simulink library "tire"  (R2020b)
settings: Solver=VariableStepAuto  StartTime=0.0  StopTime=10.0  RelTol=1e-3
undefined symbols (not defined in the file): Brakes_caliperD, Brakes_effectiveR, Brakes_kineticMu, Brakes_pads_front, Brakes_staticMu, Rim_mass, Tire_Cg, Tire_Cx, Tire_Cy, Tire_Lx, Tire_Ly, Tire_mass, Tire_muMax, Tire_muMin, Tire_prs_front, Tire_radius, Tire_VerticalK, Wheel_inertia, Wheel_width, X, Y, Z
libraries: nesl_utility x26, sm_lib x22, vehdynlibtire x2
(part 1 of 3)
settings Model: Creator=Adri  LastModifiedBy=Adri

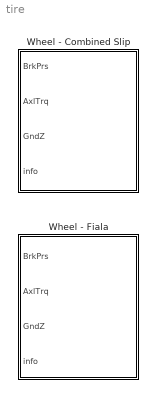
== system tire ==
  Wheel - Combined Slip : Subsystem  mask{side=Left, sideSign=1, Brake_staticMu=Brakes_staticMu, Brake_kineticMu=Brakes_kineticMu, Brake_actuatorD=Brakes_caliperD, Brake_effectiveR=Brakes_effectiveR, Brake_pads=Brakes_pads_front, Tire_radius=Tire_radius, Wheel_width=Wheel_width, Wheel_mass=Tire_mass + Rim_mass, Wheel_inertia=Wheel_inertia, Tire_prs=Tire_prs_front, Tire_verticalStiffness=Tire_VerticalK}
      mask prompts: Brake_staticMu "Static friction coefficient"; Brake_kineticMu "Kinetic friction coefficient"; Brake_actuatorD "Caliper actuator diameter"; Brake_effectiveR "Brake effective radius"; Brake_pads "Number of brake pads"; Tire_radius "Unloaded tire radius"; Wheel_width "Wheel width"; Wheel_mass "Wheel mass"; Wheel_inertia "Wheel inertia"; Tire_prs "Inflation pressure"; Tire_verticalStiffness "Vertical tire stiffness"
      settings: PortSchema="{\"entries\":[{\"content\":{\"sides\":[{\"content\":{\"connectorIds\":[\"LConn1\"]},\"type\":\"ConnectorPlacement.EquallySpacedRectSide\",\"uuid\":\"3662be25-634c-4dcf-b299-b3e3ad14fab2\"},{\"content\":{\"connectorIds\":[\"In1\",\"In2\",\"In3\",\"Out1\"],\"side\":\"RIGHT\"},\"type\":\"ConnectorPlacement.EquallySpacedRectSide\",\"uuid\":\"5eeeefc2-deff-4d04-aaf6-b6ca9cb4dfd2\"},{\"content\":{\"connectorIds\":[],\"side\":\"TOP\"},\"type\":\"ConnectorPlacement.EquallySpacedRectSide\",\"uuid\":\"9d9babff-f6dc-4e3d-b7b9-f7737e3c7694\"},{\"content\":{\"connectorIds\":[\"RConn1\"],\"side\":\"BOTTOM\"},\"type\":\"ConnectorPlacement.EquallySpacedRectSide\",\"uuid\":\"502eca10-01c6-46bc-9936-4bbe633b06d6\"}]},\"type\":\"ConnectorPlacement.EquallySpacedConnector\",\"uuid\":\"66182f26-71c7-4d18-82ec-2eaaaae22dab\"}],\"packageUris\":[\"http://schema.mathworks.com/mf0/Connector/19700101\"],\"version\":\"1.0\"}"
      mask TypeOptions side: Left | Right
      mask Callback side:
      | switch get_param(gcb,'side')
      |     case 'Left'
      |         set_param(gcb,'sideSign','1');
      |     case 'Right'
      |         set_param(gcb,'sideSign','-1');
      | end
      mask DialogControl DescGroupVar Prompt: Wheel
      mask DialogControl Container5 Prompt: Brakes
      mask DialogControl Brake_actuatorD Tooltip: (mm)
      mask DialogControl Brake_effectiveR Tooltip: (mm)
      mask DialogControl Container6 Prompt: Tires
      mask DialogControl Tire_radius Tooltip: (mm)
      mask DialogControl Wheel_width Tooltip: (mm)
      mask DialogControl Wheel_mass Tooltip: (kg)
      mask DialogControl Wheel_inertia Tooltip: (kg*m^2)
      mask DialogControl Tire_prs Tooltip: (Pa)
      mask DialogControl Tire_verticalStiffness Tooltip: (N/m)
      mask Display: image('$imagefile'); % Use "Edit Image" on toolstrip to change.
  Wheel - Fiala : Subsystem  mask{side=Left, sideSign=1, Brake_staticMu=Brakes_staticMu, Brake_kineticMu=Brakes_kineticMu, Brake_actuatorD=Brakes_caliperD, Brake_effectiveR=Brakes_effectiveR, Brake_pads=Brakes_pads_front, Tire_Cx=Tire_Cx, Tire_Cy=Tire_Cy, Tire_Cg=Tire_Cg, Tire_muKinetic=Tire_muMin, Tire_muStatic=Tire_muMax, Tire_Lx=Tire_Lx, Tire_Ly=Tire_Ly, Tire_radius=Tire_radius, Wheel_inertia=Wheel_inertia, Tire_Rdamp=0, Wheel_width=Wheel_width, Wheel_mass=Tire_mass + Rim_mass, Tire_prs=Tire_prs_front, Tire_Kz=Tire_VerticalK}
      mask prompts: Brake_staticMu "Static friction coefficient"; Brake_kineticMu "Kinetic friction coefficient"; Brake_actuatorD "Caliper actuator diameter"; Brake_effectiveR "Brake effective radius"; Brake_pads "Number of brake pads"; Tire_Cx "Longitudinal stiffness"; Tire_Cy "Lateral stiffness"; Tire_Cg "Camber stiffness"; Tire_muKinetic "Kinematic friction"; Tire_muStatic "Static friction"; Tire_Lx "Longitudinal relaxation length"; Tire_Ly "Lateral relaxation length"; Tire_radius "Unloaded tire radius"; Wheel_inertia "Wheel rotational inertia"; Tire_Rdamp "Rotational damping"; Wheel_width "Wheel width"; Wheel_mass "Wheel mass"; Tire_prs "Inflation pressure"; Tire_Kz "Vertical tire stiffness"
      settings: PortSchema="{\"entries\":[{\"content\":{\"sides\":[{\"content\":{\"connectorIds\":[\"LConn1\"]},\"type\":\"ConnectorPlacement.EquallySpacedRectSide\",\"uuid\":\"3662be25-634c-4dcf-b299-b3e3ad14fab2\"},{\"content\":{\"connectorIds\":[\"In1\",\"In2\",\"In3\",\"Out1\"],\"side\":\"RIGHT\"},\"type\":\"ConnectorPlacement.EquallySpacedRectSide\",\"uuid\":\"5eeeefc2-deff-4d04-aaf6-b6ca9cb4dfd2\"},{\"content\":{\"connectorIds\":[],\"side\":\"TOP\"},\"type\":\"ConnectorPlacement.EquallySpacedRectSide\",\"uuid\":\"9d9babff-f6dc-4e3d-b7b9-f7737e3c7694\"},{\"content\":{\"connectorIds\":[\"RConn1\"],\"side\":\"BOTTOM\"},\"type\":\"ConnectorPlacement.EquallySpacedRectSide\",\"uuid\":\"502eca10-01c6-46bc-9936-4bbe633b06d6\"}]},\"type\":\"ConnectorPlacement.EquallySpacedConnector\",\"uuid\":\"66182f26-71c7-4d18-82ec-2eaaaae22dab\"}],\"packageUris\":[\"http://schema.mathworks.com/mf0/Connector/19700101\"],\"version\":\"1.0\"}"
      mask TypeOptions side: Left | Right
      mask Callback side:
      | switch get_param(gcb,'side')
      |     case 'Left'
      |         set_param(gcb,'sideSign','1');
      |     case 'Right'
      |         set_param(gcb,'sideSign','-1');
      | end
      mask DialogControl DescGroupVar Prompt: Wheel
      mask DialogControl Container5 Prompt: Brakes
      mask DialogControl Brake_actuatorD Tooltip: (mm)
      mask DialogControl Brake_effectiveR Tooltip: (mm)
      mask DialogControl Container6 Prompt: Tires
      mask DialogControl Container7 Prompt: Longitudinal and lateral
      mask DialogControl Tire_Cx Tooltip: (N)
      mask DialogControl Tire_Cy Tooltip: (N/rad)
      mask DialogControl Tire_Cg Tooltip: (N/rad)
      mask DialogControl Tire_Lx Tooltip: (m)
      mask DialogControl Tire_Ly Tooltip: (m)
      mask DialogControl Container8 Prompt: Rolling
      mask DialogControl Tire_radius Tooltip: (mm)
      mask DialogControl Wheel_inertia Tooltip: (kg*m^2)
      mask DialogControl Tire_Rdamp Tooltip: (N*m)/(rad/s)
      mask DialogControl Container12 Prompt: Aligning
      mask DialogControl Wheel_width Tooltip: (mm)
      mask DialogControl Container11 Prompt: Vertical
      mask DialogControl Wheel_mass Tooltip: (kg)
      mask DialogControl Tire_prs Tooltip: (Pa)
      mask DialogControl Tire_Kz Tooltip: (N/m)
      mask Display: image('$imagefile'); % Use "Edit Image" on toolstrip to change.

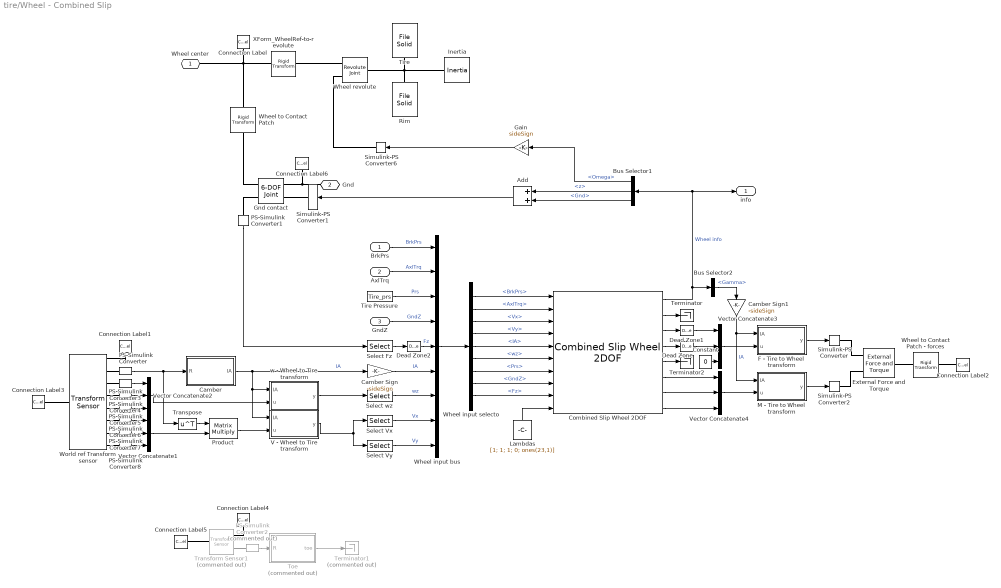
== system tire/Wheel - Combined Slip ==
  BrkPrs : Inport
  AxlTrq : Inport  Port=2
  GndZ : Inport  Port=3
  Add : Sum
  Bus Selector1 : BusSelector  OutputSignals=Omega,z,Gnd
  Bus Selector2 : BusSelector  OutputSignals=Gamma
  Camber : MATLAB Function  TreatAsAtomicUnit=on
  Camber Sign : Gain  Gain=-sideSign
  Camber Sign1 : Gain  Gain=-sideSign
  Combined Slip Wheel 2DOF : vehdynlibtire/Combined Slip Wheel 2DOF  BrakeType=Disc  mu_static=Brake_staticMu  mu_kinetic=Brake_kineticMu  disk_abore=Brake_actuatorD*1e-3  Rm=Brake_effectiveR*1e-3  num_pads=Brake_pads  drum_abore=0.0508  drum_a=0.123  drum_c=0.212  drum_r=0.15  drum_theta1=0  drum_theta2=126  brake_p_bpt=[1 11.4736842105263 21.9473684210526 32.4210526315789 42.8947368421053 53.3684210526316 63.8421052631579 74.3157894736842 84.7894736842105 95.2631578947368 105.736842105263 116.210526315789 126.684210526316 137.157894736842 147.631578947368 158.105263157895 168.578947368421 179.052631578947 189.526315789474 200]  brake_n_bpt=[0 52.6315789473684 105.263157894737 157.894736842105 210.526315789474 263.157894736842 315.789473684211 368.421052631579 421.052631578947 473.684210526316 526.315789473684 578.947368421053 631.578947368421 684.210526315789 736.842105263158 789.473684210526 842.105263157895 894.736842105263 947.368421052632 1000]  f_brake_t=[43.4900602404453 42.5056030554862 41.5350898940194 40.5780454442085 39.6340111501808 38.7025443887544 37.7832176914519 36.8756180088306 35.9793460143796 35.0940154454303 34.2192524787115 33.3546951383474 32.4999927342521 31.6548053290159 30.8188032315107 29.991666515561 29.1730845621415 28.362755623661 27.5603864089927 26.765691687993;498.991217495636 487.695866636631 476.560505099801 465.579679307235 454.748127933653 444.060772460445 433.51270824929 423.099196101319 412.81565427025 402.657650900201 392.620896861006 382.701238955775 372.894653477208 363.197240090814 353.605216024701 344.114910546964 334.722759712992 325.425301366216 316.219170376863 307.10109410434;954.492374750826 932.886130217776 911.585920305583 890.581313170261 869.862244717126 849.419000532136 829.242198807128 809.322774193808 789.651962526121 770.221286354971 751.0225412433 732.047782773203 713.289314220164 694.739674852612 676.391628817892 658.238154578366 640.272434863842 622.48784710877 604.877954344734 587.436496520688;1409.99353200602 1378.07639379892 1346.61133551136 1315.58294703329 1284.9763615006 1254.77722860383 1224.97168936497 1195.5463522863 1166.48827078199 1137.78492180974 1109.42418562559 1081.39432659063 1053.68397496312 1026.28210961441 999.178041611083 972.361398609768 945.822110014692 919.550392851325 893.536738312604 867.771898937035;1865.49468926121 1823.26665738007 1781.63675071715 1740.58458089631 1700.09047828407 1660.13545667552 1620.7011799228 1581.76993037878 1543.32457903786 1505.34855726451 1467.82583000789 1430.74087040806 1394.07863570608 1357.82454437621 1321.96445440427 1286.48464264117 1251.37178516554 1216.61293859388 1182.19552228048 1148.10730135338;2320.9958465164 2268.45692096121 2216.66216592293 2165.58621475934 2115.20459506754 2065.49368474721 2016.43067048064 1967.99350847127 1920.16088729373 1872.91219271928 1826.22747439018 1780.08741422549 1734.47329644903 1689.36697913801 1644.75086719747 1600.60788667257 1556.92146031639 1513.67548433643 1470.85430624835 1428.44270376973;2776.49700377159 2713.64718454235 2651.68758112871 2590.58784862237 2530.31871185102 2470.8519128189 2412.16016103848 2354.21708656376 2296.9971955496 2240.47582817405 2184.62911877248 2129.43395804292 2074.86795719199 2020.9094138998 1967.53727999066 1914.73113070398 1862.47113546724 1810.73803007899 1759.51309021622 1708.77810618608;3231.99816102678 3158.8374481235 3086.71299633449 3015.58948248539 2945.43282863449 2876.21014089059 2807.88965159632 2740.44066465625 2673.83350380547 2608.03946362882 2543.03076315477 2478.78050186034 2415.26261793494 2352.4518486616 2290.32369278385 2228.85437473538 2168.02081061809 2107.80057582154 2048.17187418409 1989.11350860242;3687.49931828197 3604.02771170464 3521.73841154027 3440.59111634842 3360.54694541796 3281.56836896228 3203.61914215416 3126.66424274874 3050.66981206134 2975.60309908359 2901.43240753707 2828.12704567777 2755.6572786779 2683.9942834234 2613.11010557704 2542.97761876678 2473.57048576894 2404.8631215641 2336.83065815196 2269.44891101877;4143.00047553716 4049.21797528579 3956.76382674606 3865.59275021144 3775.66106220143 3686.92659703397 3599.34863271199 3512.88782084123 3427.50612031721 3343.16673453836 3259.83405191936 3177.4735894952 3096.05193942085 3015.5367181852 2935.89651837023 2857.10086279818 2779.12016091979 2701.92566730665 2625.48944211983 2549.78431343512;4598.50163279235 4494.40823886693 4391.78924195184 4290.59438407447 4190.77517898491 4092.28482510566 3995.07812326983 3899.11139893372 3804.34242857308 3710.73036999313 3618.23569630166 3526.82013331263 3436.44660016381 3347.079152947 3258.68293116342 3171.22410682959 3084.66983607064 2998.98821304921 2914.1482260877 2830.11971585147;5054.00279004754 4939.59850244808 4826.81465715762 4715.59601793749 4605.88929576838 4497.64305317735 4390.80761382767 4285.3349770262 4181.17873682896 4078.2940054479 3976.63734068395 3876.16667713006 3776.84126090677 3678.62158770879 3581.46934395661 3485.34735086099 ...(+2764 chars)]  tireParamSet=vdynPassCar.mat  plySteer=off  turnslip=off  PRESMAX=1003118  PRESMIN=9982  FZMAX=3500  FZMIN=100  VXLOW=0.5  KPUMAX=2  KPUMIN=-2  ALPMAX=1.5708  ALPMIN=-1.5708  CAMMAX=0.173142086627737  CAMMIN=-0.173348165334087  LONGVL=16.7  omegao=0  br=1e-3  UNLOADED_RADIUS=Tire_radius*1e-3  NOMPRES=1e5  FNOMIN=750  WIDTH=Wheel_width*1e-3  RIM_RADIUS=.19  MASS=Wheel_mass  IYY=Wheel_inertia(3)  GRAVITY=-9.80665  zo=0  zdoto=0  BREFF=8.25094594147963  DREFF=0.260468730454265  FREFF=0.0735298544471851  Q_RE0=1.00866439868088  Q_V1=0.000760413786224011  Q_V2=0.0463384792019201  Q_FZ1=0  Q_FZ2=15.6870832810226  Q_FZ3=0  Q_FCX=0.138643970247602  Q_FCY=0.10843499565426  Q_FCY2=-0.465763352339538  PFZ1=0.69958166705601  VERTICAL_STIFFNESS=Tire_verticalStiffness  VERTICAL_DAMPING=494.649255786991  BOTTOM_OFFST=.01  BOTTOM_STIFF=2e6  LONGITUDINAL_STIFFNESS=388714.175879854  LATERAL_STIFFNESS=157087.404633332  PCFX1=0.18539229191199  PCFX2=0  PCFX3=0  PCFY1=0.163183345037677  PCFY2=0  PCFY3=0.249094918231954  Q_RA1=0.675942571700787  Q_RA2=0.73800463546164  Q_RB1=1.04487486456705  Q_RB2=-1.191763806629  PCX1=1.58523057950359  PDX1=1.0239116238178  PDX2=-0.0842405110022724  PDX3=0  PEX1=0.110312777158455  PEX2=0.313468516038146  PEX3=0  PEX4=0.0016060905760045  PKX1=21.3872544684023  PKX2=14.0006541873175  PKX3=-0.405326109653452  PHX1=0.000212599305364818  PHX2=0.00115950515263055  PVX1=1.59236164471432e-05  PVX2=0.000104321112127671  PPX1=-0.349461321276586  PPX2=0.387840040616429  PPX3=-0.0969947336569324  PPX4=0.0632271859795801  RBX1=12.7633329850276  RBX2=9.5787123658471  RBX3=0  RCX1=1.02796280922059  REX1=-0.45202516851367  REX2=-0.47304886171176  RHX1=0.000233272373115809  QSX1=-0.00788307788961443  QSX2=0.954629515459396  QSX3=0.0155855777667025  QSX4=0.125904607142414  QSX5=1.01110069703963  QSX6=20.1938577118433  QSX7=0.310818120717083  QSX8=-0.0430823751139655  QSX9=0.636494404888216  QSX10=0.142438060591663  QSX11=0.346766530036373  QSX12=0  QSX13=0  QSX14=0  PPMX1=0  PCY1=1.34299950037631  PDY1=0.878267729082195  PDY2=-0.0644597923147385  PDY3=0  PEY1=-0.809776534470972  PEY2=-0.600180598867198  PEY3=0.0991732552633487  PEY4=-6.5577974035573  PEY5=0  PKY1=-15.5714726518315  PKY2=1.73126522291751  PKY3=0.365349873517229  PKY4=1.98176755955416  PKY5=0  PKY6=-0.884005199550313  PKY7=-0.237259727611847  PHY1=-0.00183370557235628  PHY2=0.00346401302716671  PVY1=-0.00675427560163264  PVY2=0.036379218103843  PVY3=-0.163543984089166  PVY4=-0.491003349625726  PPY1=-0.62059646553185  PPY2=-0.0647824842338686  PPY3=-0.164648843290686  PPY4=0.283193909060098  PPY5=0  RBY1=10.7588809173639  RBY2=7.70420065295029  RBY3=3.40283755070691e-06  RBY4=0  RCY1=1.06691874059059  REY1=0.308244924574305  REY2=7.48775032604508e-06  RHY1=0.0118479204960415  RHY2=7.63650177161071e-06  RVY1=0.0560024425050078  RVY2=7.48487127056197e-06  RVY3=0  RVY4=98.4047026517149  RVY5=2.02759273900054  RVY6=15.7623064923347  QSY1=0.00699077564863536  QSY2=0  QSY3=0.00153535478298811  QSY4=8.55710322455322e-05  QSY5=0  QSY6=0  QSY7=0.89443879773793  QSY8=-0.403227641260894  QBZ1=11.666656027484  QBZ2=-1.30355438574485  QBZ3=0  QBZ4=0.177918305399071  QBZ5=-0.162481135068033  QBZ6=0  QBZ9=30.1445534682089  QBZ10=0  QCZ1=1.29026978207574  QDZ1=0.0886972644991399  QDZ2=-0.0058634820161856  QDZ3=0.3805597481383  QDZ4=0  QDZ6=0.00160914918118959  QDZ7=-0.00211036330862154  QDZ8=-0.13921904912557  QDZ9=0.00816585550028243  QDZ10=0  QDZ11=0  QEZ1=-2.19802254534746  QEZ2=1.01850535789165  QEZ3=0  QEZ4=0.278379679112054  QEZ5=-0.548414722765386  QHZ1=0.00148361198869669  QHZ2=0.00202017567585904  QHZ3=0.240316641332066  QHZ4=-0.210114035738085  PPZ1=-0.443927982388615  PPZ2=0  SSZ1=0.00914999585397887  SSZ2=0.0389830656052735  SSZ3=0  SSZ4=0  PDXP1=0.396718274678791  PDXP2=0  PDXP3=0  PKYP1=1.00587060633573  PDYP1=0.40483048923438  PDYP2=0  PDYP3=0  PDYP4=0  PHYP1=0.992731942067188  PHYP2=0.150352945499914  PHYP3=0  PHYP4=-3.98988682633674  PECP1=0.502379254513503  PECP2=0  QDTP1=10.0178654287947  QCRP1=0.200627747200702  QCRP2=0.0995735881599772  QBRP1=0.0997107127960717  QDRP1=1.01432910167423  QDRP2=0  aMode=2
      link override Magic Tire Const Input/Fx Relaxation/Integrator: AbsoluteTolerance=1e-2
      link override Magic Tire Const Input/Fy Relaxation/Integrator: AbsoluteTolerance=1e-2
      link override Magic Tire Const Input/My Relaxation/Integrator: AbsoluteTolerance=1e-2
      settings: SourceProductBaseCode=VE
  Connection Label{,1..2,4} (4 alike) : ConnectionLabel  Label=WheelRef
  Connection Label3 : ConnectionLabel  Label=GroundRef
  Connection Label5 : ConnectionLabel  Label=ChassisRef
  Connection Label6 : ConnectionLabel  Label=GroundRef
  Constant : Constant  Value=0
  Dead Zone : DeadZone  LowerValue=-10  UpperValue=10  ZeroCross=off  SaturateOnIntegerOverflow=on
  Dead Zone1 : DeadZone  LowerValue=-1  UpperValue=1  ZeroCross=off  SaturateOnIntegerOverflow=on
  Dead Zone2 : DeadZone  LowerValue=-inf  UpperValue=0  ZeroCross=off  SaturateOnIntegerOverflow=on
  External Force and Torque : sm_lib/Forces and Torques/External Force and Torque  ForceResolutionFrame=AttachedFrame  EnableForceX=off  EnableForceY=off  EnableForceZ=off  EnableForce=on  TorqueResolutionFrame=AttachedFrame  EnableTorqueX=off  EnableTorqueY=off  EnableTorqueZ=off  EnableTorque=on
  F - Tire to Wheel transform : MATLAB Function  TreatAsAtomicUnit=on
  Gain : Gain  Gain=sideSign
  Gnd contact : sm_lib/Joints/6-DOF Joint  JointMode=Normal  SenseConstraintForce=off  SenseConstraintForceX=off  SenseConstraintForceY=off  SenseConstraintForceZ=off  SenseConstraintTorque=off  SenseConstraintTorqueX=off  SenseConstraintTorqueY=off  SenseConstraintTorqueZ=off  SenseTotalForce=on  SenseTotalForceX=off  SenseTotalForceY=off  SenseTotalForceZ=off  SenseTotalTorque=off  SenseTotalTorqueX=off  SenseTotalTorqueY=off  SenseTotalTorqueZ=off  CompositeWrenchDir=BaseOnFollower  CompositeWrenchFrame=BaseFrame  PxEquilibriumPosition=0  PxEquilibriumPositionUnits=m  PxSpringStiffness=0  PxSpringStiffnessUnits=N/m  PxDampingCoefficient=0  PxDampingCoefficientUnits=N/(m/s)  PxTorqueActuationMode=NoTorque  PxMotionActuationMode=ComputedMotion  PxSensePosition=off  PxSenseVelocity=off  PxSenseAcceleration=off  PxSenseTorqueForce=off  PxSenseLowerLimitTorqueForce=off  PxSenseUpperLimitTorqueForce=off  PxLowerLimitSpecify=off  PxLowerLimitBound=-1  PxLowerLimitBoundUnits=m  PxLowerLimitStiffness=1e6  PxLowerLimitStiffnessUnits=N/m  PxLowerLimitDamping=1e3  PxLowerLimitDampingUnits=N/(m/s)  PxLowerLimitTransitionRegionWidth=1e-4  PxLowerLimitTransitionRegionWidthUnits=m  PxUpperLimitSpecify=off  PxUpperLimitBound=1  PxUpperLimitBoundUnits=m  PxUpperLimitStiffness=1e6  PxUpperLimitStiffnessUnits=N/m  PxUpperLimitDamping=1e3  PxUpperLimitDampingUnits=N/(m/s)  PxUpperLimitTransitionRegionWidth=1e-4  PxUpperLimitTransitionRegionWidthUnits=m  PxPositionTargetSpecify=off  PxPositionTargetPriority=Low  PxPositionTargetValue=-500  PxPositionTargetValueUnits=mm  PxVelocityTargetSpecify=off  PxVelocityTargetPriority=High  PxVelocityTargetValue=0  PxVelocityTargetValueUnits=m/s  PyEquilibriumPosition=0  PyEquilibriumPositionUnits=m  PySpringStiffness=0  PySpringStiffnessUnits=N/m  PyDampingCoefficient=0  PyDampingCoefficientUnits=N/(m/s)  PyTorqueActuationMode=NoTorque  PyMotionActuationMode=ComputedMotion  PySensePosition=off  PySenseVelocity=off  PySenseAcceleration=off  PySenseTorqueForce=off  PySenseLowerLimitTorqueForce=off  PySenseUpperLimitTorqueForce=off  PyLowerLimitSpecify=off  PyLowerLimitBound=-1  PyLowerLimitBoundUnits=m  PyLowerLimitStiffness=1e6  PyLowerLimitStiffnessUnits=N/m  PyLowerLimitDamping=1e3  PyLowerLimitDampingUnits=N/(m/s)  PyLowerLimitTransitionRegionWidth=1e-4  PyLowerLimitTransitionRegionWidthUnits=m  PyUpperLimitSpecify=off  PyUpperLimitBound=1  PyUpperLimitBoundUnits=m  PyUpperLimitStiffness=1e6  PyUpperLimitStiffnessUnits=N/m  PyUpperLimitDamping=1e3  PyUpperLimitDampingUnits=N/(m/s)  PyUpperLimitTransitionRegionWidth=1e-4  PyUpperLimitTransitionRegionWidthUnits=m  PyPositionTargetSpecify=off  PyPositionTargetPriority=Low  PyPositionTargetValue=600*sideSign  PyPositionTargetValueUnits=mm  PyVelocityTargetSpecify=off  PyVelocityTargetPriority=High  PyVelocityTargetValue=0  PyVelocityTargetValueUnits=m/s  PzEquilibriumPosition=0  PzEquilibriumPositionUnits=m  PzSpringStiffness=0  PzSpringStiffnessUnits=N/m  PzDampingCoefficient=0  PzDampingCoefficientUnits=N/(m/s)  PzTorqueActuationMode=ComputedTorque  PzMotionActuationMode=InputMotion  PzSensePosition=off  PzSenseVelocity=off  PzSenseAcceleration=off  PzSenseTorqueForce=off  PzSenseLowerLimitTorqueForce=off  PzSenseUpperLimitTorqueForce=off  PzLowerLimitSpecify=off  PzLowerLimitBound=-1  PzLowerLimitBoundUnits=m  PzLowerLimitStiffness=1e6  PzLowerLimitStiffnessUnits=N/m  PzLowerLimitDamping=1e3  PzLowerLimitDampingUnits=N/(m/s)  PzLowerLimitTransitionRegionWidth=1e-4  PzLowerLimitTransitionRegionWidthUnits=m  PzUpperLimitSpecify=off  PzUpperLimitBound=1  PzUpperLimitBoundUnits=m  PzUpperLimitStiffness=1e6  PzUpperLimitStiffnessUnits=N/m  PzUpperLimitDamping=1e3  PzUpperLimitDampingUnits=N/(m/s)  PzUpperLimitTransitionRegionWidth=1e-4  PzUpperLimitTransitionRegionWidthUnits=m  PzPositionTargetSpecify=on  PzPositionTargetPriority=High  PzPositionTargetValue=0  PzPositionTargetValueUnits=m  PzVelocityTargetSpecify=off  PzVelocityTargetPriority=High  PzVelocityTargetValue=0  PzVelocityTargetValueUnits=m/s  SphDefPosRotationMethod=None  SphDefPosRotationAngleUnits=deg  SphDefPosRotationStandardAxis=+Z  SphDefPosRotationAngle=0.0  SphDefPosRotationArbitraryAxis=[0 0 1]  SphDefPosFollAlignAxisA=+X  SphDefPosBaseAlignAxisA=+Y  SphDefPosFollAlignAxisB=+Y  SphDefPosBaseAlignAxisB=+Z  SphDefPosRotationSequenceAxes=FollowerAxes  SphDefPosRotationSequence=XYX  SphDefPosRotationSequenceAngles=[0 0 0]  SphDefPosRotationSequenceAnglesUnits=deg  SphDefPosRotationMatrix=[1 0 0; 0 1 0; 0 0 1]  SphEqPosRotationMethod=None  SphEqPosRotationAngleUnits=deg  SphEqPosRotationStandardAxis=+Z  SphEqPosRotationAngle=0.0  SphEqPosRotationArbitraryAxis=[0 0 1]  SphEqPosFollAlignAxisA=+X  SphEqPosBaseAlignAxisA=+Y  SphEqPosFollAlignAxisB=+Y  SphEqPosBaseAlignAxisB=+Z  SphEqPosRotationSequenceAxes=FollowerAxes  SphEqPosRotationSequence=XYX  SphEqPosRotationSequenceAngles=[0 0 0]  SphEqPosRotationSequenceAnglesUnits=deg  SphEqPosRotationMatrix=[1 0 0; 0 1 0; 0 0 1]  SphSpringStiffness=0  SphSpringStiffnessUnits=N*m/deg  SphDampingCoefficient=0  SphDampingCoefficientUnits=N*m/(deg/s)  SphActuateTorqueX=off  SphActuateTorqueY=off  SphActuateTorqueZ=off  SphActuateTorque=off  SphTorqueActuationMode=NoTorque  SphMotionActuationMode=ComputedMotion  SphActuationFrame=BaseFrame  SphSensePosition=off  SphSenseVelocityX=off  SphSenseVelocityY=off  SphSenseVelocityZ=off  SphSenseVelocity=off  SphSenseAccelerationX=off  SphSenseAccelerationY=off  SphSenseAccelerationZ=off  SphSenseAcceleration=off  SphSenseTorqueX=off  SphSenseTorqueY=off  SphSenseTorqueZ=off  SphSenseTorqueForce=off  SphSenseLowerLimitTorqueMag=off  SphSenseUpperLimitTorqueMag=off  SphSensingFrame=BaseFrame  SphLowerLimitSpecify=off  SphLowerLimitBound=15  SphLowerLimitBoundUnits=deg  SphLowerLimitStiffness=1e4  SphLowerLimitStiffnessUnits=N*m/deg  SphLowerLimitDamping=10  SphLowerLimitDampingUnits=N*m/(deg/s)  SphLowerLimitTransitionRegionWidth=0.1  SphLowerLimitTransitionRegionWidthUnits=deg  SphUpperLimitSpecify=off  SphUpperLimitBound=45  SphUpperLimitBoundUnits=deg  SphUpperLimitStiffness=1e4  SphUpperLimitStiffnessUnits=N*m/deg  SphUpperLimitDamping=10  SphUpperLimitDampingUnits=N*m/(deg/s)  SphUpperLimitTransitionRegionWidth=0.1  SphUpperLimitTransitionRegionWidthUnits=deg  SphPositionTargetRotationMethod=AlignedAxes  SphPositionTargetRotationAngleUnits=deg  SphPositionTargetRotationStandardAxis=+Z  SphPositionTargetRotationAngle=0.0  SphPositionTargetRotationArbitraryAxis=[0 0 1]  SphPositionTargetFollAlignAxisA=+Z  SphPositionTargetBaseAlignAxisA=+Z  SphPositionTargetFollAlignAxisB=+X  SphPositionTargetBaseAlignAxisB=+X  SphPositionTargetRotationSequenceAxes=FollowerAxes  SphPositionTargetRotationSequence=XYX  SphPositionTargetRotationSequenceAngles=[0 0 0]  SphPositionTargetRotationSequenceAnglesUnits=deg  SphPositionTargetRotationMatrix=[1 0 0; 0 1 0; 0 0 1]  SphPositionTargetSpecify=on  SphPositionTargetPriority=Low  SphVelocityTargetValue=[0 0 0]  SphVelocityTargetValueUnits=deg/s  SphVelocityTargetSpecify=off  SphVelocityTargetPriority=High  SphVelocityTargetInFollowerFrame=on
  Inertia : sm_lib/Body Elements/Inertia  InertiaType=Custom  Mass=Wheel_mass  MassUnits=kg  CenterOfMass=[0 0 0]  CenterOfMassUnits=m  MomentsOfInertia=Wheel_inertia  MomentsOfInertiaUnits=kg*m^2  ProductsOfInertia=[0 0 0]  ProductsOfInertiaUnits=kg*m^2  GraphicType=None  MarkerShape=Inertia  MarkerSize=20  GraphicVisPropType=SimpleVisualProperties  GraphicDiffuseColor=[0.5 0.5 0.5]  GraphicSpecularColor=[0.5 0.5 0.5 1.0]  GraphicAmbientColor=[0.15 0.15 0.15 1.0]  GraphicEmissiveColor=[0.0 0.0 0.0 1.0]  GraphicShininess=75  GraphicOpacity=1.0
  Lambdas : Constant  Value=[1; 1; 1; 0; ones(23,1)]
  M - Tire to Wheel transform : MATLAB Function  TreatAsAtomicUnit=on
  PS-Simulink Converter{,3..8} (7 alike) : nesl_utility/PS-Simulink Converter  PhysicalDomain=network_engine_domain  SubClassName=ps_output  LeftPortType=input  RightPortType=output  PseudoPeriodic=off  Frequencies=[]  Unit=inherit  AffineConversion=off
  PS-Simulink Converter1 : nesl_utility/PS-Simulink Converter  PhysicalDomain=network_engine_domain  SubClassName=ps_output  LeftPortType=input  RightPortType=output  PseudoPeriodic=off  Frequencies=[]  Unit=N  AffineConversion=off
  PS-Simulink Converter2 : nesl_utility/PS-Simulink Converter  Commented=on  PhysicalDomain=network_engine_domain  SubClassName=ps_output  LeftPortType=input  RightPortType=output  PseudoPeriodic=off  Frequencies=[]  Unit=inherit  AffineConversion=off
  Product : Product  Multiplication=Matrix(*)
  Rim : sm_lib/Body Elements/File Solid  ExtGeomFileName=.\CAD\WT_80101.stp  UnitType=FromFile  ExtGeomFileUnits=m  StepReaderType=HEX  ExportConvexHullGeometry=off  InertiaType=CalculateFromGeometry  Mass=1  MassUnits=g  CenterOfMass=[0 0 0]  CenterOfMassUnits=m  MomentsOfInertia=[1 1 1]  MomentsOfInertiaUnits=kg*m^2  ProductsOfInertia=[0 0 0]  ProductsOfInertiaUnits=kg*m^2  BasedOnType=Mass  Density=689.8  DensityUnits=kg/m^3  DoExposeReferenceFrame=on  SerializedFrames=<Frames/>  GraphicType=FromGeometry  MarkerShape=Sphere  MarkerSize=10  GraphicVisPropType=SimpleVisualProperties  GraphicDiffuseColor=[0.4 0.4 0.4]  GraphicSpecularColor=[0.5 0.5 0.5 1.0]  GraphicAmbientColor=[0.15 0.15 0.15 1.0]  GraphicEmissiveColor=[0.0 0.0 0.0 1.0]  GraphicShininess=75  GraphicOpacity=1.0
  Select Fz : Selector  InputPortWidth=3  IndexOptions=Index vector (dialog)  Indices=3  OutputSizes=1
  Select Vx : Selector  InputPortWidth=3  IndexOptions=Index vector (dialog)  Indices=1  OutputSizes=1
  Select Vy : Selector  InputPortWidth=3  IndexOptions=Index vector (dialog)  Indices=2  OutputSizes=1
  Select wz : Selector  InputPortWidth=3  IndexOptions=Index vector (dialog)  Indices=3  OutputSizes=1
  Simulink-PS Converter : nesl_utility/Simulink-PS Converter  PhysicalDomain=network_engine_domain  SubClassName=ps_input  LeftPortType=input  RightPortType=output  PseudoPeriodic=off  Frequencies=[]  NoiseDistribution=none  NoiseParameters=[]  Unit=N  AffineConversion=off  FilteringAndDerivatives=provide  SimscapeFilterOrder=1  InputFilterTimeConstant=0.001  UdotUserProvided=0
  Simulink-PS Converter1 : nesl_utility/Simulink-PS Converter  PhysicalDomain=network_engine_domain  SubClassName=ps_input  LeftPortType=input  RightPortType=output  PseudoPeriodic=off  Frequencies=[]  NoiseDistribution=none  NoiseParameters=[]  Unit=m  AffineConversion=off  FilteringAndDerivatives=filter  SimscapeFilterOrder=2  InputFilterTimeConstant=0.1  UdotUserProvided=0
  Simulink-PS Converter2 : nesl_utility/Simulink-PS Converter  PhysicalDomain=network_engine_domain  SubClassName=ps_input  LeftPortType=input  RightPortType=output  PseudoPeriodic=off  Frequencies=[]  NoiseDistribution=none  NoiseParameters=[]  Unit=N*m  AffineConversion=off  FilteringAndDerivatives=provide  SimscapeFilterOrder=1  InputFilterTimeConstant=0.001  UdotUserProvided=0
  Simulink-PS Converter6 : nesl_utility/Simulink-PS Converter  PhysicalDomain=network_engine_domain  SubClassName=ps_input  LeftPortType=input  RightPortType=output  PseudoPeriodic=off  Frequencies=[]  NoiseDistribution=none  NoiseParameters=[]  Unit=rad  AffineConversion=off  FilteringAndDerivatives=filter  SimscapeFilterOrder=2  InputFilterTimeConstant=0.2  UdotUserProvided=0
  Terminator : Terminator
  Terminator1 : Terminator  Commented=on
  Terminator2 : Terminator
  Tire : sm_lib/Body Elements/File Solid  ExtGeomFileName=.\CAD\WT_80102.stp  UnitType=FromFile  ExtGeomFileUnits=m  StepReaderType=HEX  ExportConvexHullGeometry=off  InertiaType=CalculateFromGeometry  Mass=1  MassUnits=g  CenterOfMass=[0 0 0]  CenterOfMassUnits=m  MomentsOfInertia=[1 1 1]  MomentsOfInertiaUnits=kg*m^2  ProductsOfInertia=[0 0 0]  ProductsOfInertiaUnits=kg*m^2  BasedOnType=Mass  Density=910  DensityUnits=kg/m^3  DoExposeReferenceFrame=on  SerializedFrames=<Frames/>  GraphicType=FromGeometry  MarkerShape=Sphere  MarkerSize=10  GraphicVisPropType=SimpleVisualProperties  GraphicDiffuseColor=[0.2 0.2 0.2]  GraphicSpecularColor=[0.5 0.5 0.5 1.0]  GraphicAmbientColor=[0.15 0.15 0.15 1.0]  GraphicEmissiveColor=[0.0 0.0 0.0 1.0]  GraphicShininess=75  GraphicOpacity=1.0
  Tire Pressure : Constant  Value=Tire_prs
  Toe : MATLAB Function  Commented=on  TreatAsAtomicUnit=on
  Transform Sensor1 : sm_lib/Frames and Transforms/Transform Sensor  Commented=on  MeasurementFrame=World  SenseAngle=off  SenseAxis=off  SenseAngle1=off  SenseAngle2=off  SenseAngle3=off  SenseQ=off  SenseR=on  SenseOmegaX=off  SenseOmegaY=off  SenseOmegaZ=off  SenseOmega1=off  SenseOmega2=off  SenseOmega3=off  SenseQDot=off  SenseRDot=off  SenseAlphaX=off  SenseAlphaY=off  SenseAlphaZ=off  SenseAlpha1=off  SenseAlpha2=off  SenseAlpha3=off  SenseQDDot=off  SenseRDDot=off  SenseX=off  SenseY=off  SenseZ=off  SenseRad=off  SenseAzim=off  SenseDist=off  SenseInc=off  SenseXDot=off  SenseYDot=off  SenseZDot=off  SenseRadDot=off  SenseAzimDot=off  SenseDistDot=off  SenseIncDot=off  SenseXDDot=off  SenseYDDot=off  SenseZDDot=off  SenseRadDDot=off  SenseAzimDDot=off  SenseDistDDot=off  SenseIncDDot=off
  Transpose : Math  Operator=transpose  SaturateOnIntegerOverflow=on
  V - Wheel to Tire transform : MATLAB Function  TreatAsAtomicUnit=on
  Vector Concatenate{1..4} (4 alike) : Concatenate  NumInputs=3
  Wheel input bus : BusCreator  Inputs=9
  Wheel input selecto : BusSelector  OutputSignals=BrkPrs,AxlTrq,Vx,Vy,IA,wz,Prs,GndZ,Fz
  Wheel revolute : sm_lib/Joints/Revolute Joint  JointMode=Normal  SenseConstraintForce=off  SenseConstraintForceX=off  SenseConstraintForceY=off  SenseConstraintForceZ=off  SenseConstraintTorque=off  SenseConstraintTorqueX=off  SenseConstraintTorqueY=off  SenseConstraintTorqueZ=off  SenseTotalForce=off  SenseTotalForceX=off  SenseTotalForceY=off  SenseTotalForceZ=off  SenseTotalTorque=off  SenseTotalTorqueX=off  SenseTotalTorqueY=off  SenseTotalTorqueZ=off  CompositeWrenchDir=FollowerOnBase  CompositeWrenchFrame=BaseFrame  EquilibriumPosition=0  EquilibriumPositionUnits=deg  SpringStiffness=0  SpringStiffnessUnits=N*m/deg  DampingCoefficient=0  DampingCoefficientUnits=N*m/(deg/s)  TorqueActuationMode=ComputedTorque  MotionActuationMode=InputMotion  SensePosition=off  SenseVelocity=off  SenseAcceleration=off  SenseTorqueForce=off  SenseLowerLimitTorqueForce=off  SenseUpperLimitTorqueForce=off  LowerLimitSpecify=off  LowerLimitBound=-90  LowerLimitBoundUnits=deg  LowerLimitStiffness=1e4  LowerLimitStiffnessUnits=N*m/deg  LowerLimitDamping=10  LowerLimitDampingUnits=N*m/(deg/s)  LowerLimitTransitionRegionWidth=0.1  LowerLimitTransitionRegionWidthUnits=deg  UpperLimitSpecify=off  UpperLimitBound=90  UpperLimitBoundUnits=deg  UpperLimitStiffness=1e4  UpperLimitStiffnessUnits=N*m/deg  UpperLimitDamping=10  UpperLimitDampingUnits=N*m/(deg/s)  UpperLimitTransitionRegionWidth=0.1  UpperLimitTransitionRegionWidthUnits=deg  PositionTargetSpecify=off  PositionTargetPriority=High  PositionTargetValue=0  PositionTargetValueUnits=deg  VelocityTargetSpecify=off  VelocityTargetPriority=High  VelocityTargetValue=0  VelocityTargetValueUnits=deg/s
  Wheel to Contact Patch : sm_lib/Frames and Transforms/Rigid Transform  TranslationMethod=StandardAxis  TranslationStandardOffset=Tire_radius  TranslationLengthUnit=mm  TranslationStandardAxis=-Z  TranslationCartesianOffset=[0 0 0]  TranslationROffset=0  TranslationROffsetUnits=m  TranslationZOffset=0  TranslationZOffsetUnits=m  TranslationThetaOffset=0  TranslationThetaOffsetUnits=deg  RotationMethod=None  RotationAngleUnits=deg  RotationStandardAxis=+Z  RotationAngle=0.0  RotationArbitraryAxis=[0 0 1]  FollAlignAxisA=+Z  BaseAlignAxisA=-X  FollAlignAxisB=+Y  BaseAlignAxisB=+Z  RotationSequenceAxes=FollowerAxes  RotationSequence=XYX  RotationSequenceAngles=[0 0 0]  RotationSequenceAnglesUnits=deg  RotationMatrix=[1 0 0; 0 1 0; 0 0 1]
  Wheel to Contact Patch - forces : sm_lib/Frames and Transforms/Rigid Transform  TranslationMethod=StandardAxis  TranslationStandardOffset=Tire_radius  TranslationLengthUnit=mm  TranslationStandardAxis=-Z  TranslationCartesianOffset=[0 0 0]  TranslationROffset=0  TranslationROffsetUnits=m  TranslationZOffset=0  TranslationZOffsetUnits=m  TranslationThetaOffset=0  TranslationThetaOffsetUnits=deg  RotationMethod=None  RotationAngleUnits=deg  RotationStandardAxis=+Z  RotationAngle=0.0  RotationArbitraryAxis=[0 0 1]  FollAlignAxisA=+Z  BaseAlignAxisA=-X  FollAlignAxisB=+Y  BaseAlignAxisB=+Z  RotationSequenceAxes=FollowerAxes  RotationSequence=XYX  RotationSequenceAngles=[0 0 0]  RotationSequenceAnglesUnits=deg  RotationMatrix=[1 0 0; 0 1 0; 0 0 1]
  World ref Transform sensor : sm_lib/Frames and Transforms/Transform Sensor  MeasurementFrame=World  SenseAngle=off  SenseAxis=off  SenseAngle1=off  SenseAngle2=off  SenseAngle3=off  SenseQ=off  SenseR=on  SenseOmegaX=on  SenseOmegaY=on  SenseOmegaZ=on  SenseOmega1=off  SenseOmega2=off  SenseOmega3=off  SenseQDot=off  SenseRDot=off  SenseAlphaX=off  SenseAlphaY=off  SenseAlphaZ=off  SenseAlpha1=off  SenseAlpha2=off  SenseAlpha3=off  SenseQDDot=off  SenseRDDot=off  SenseX=off  SenseY=off  SenseZ=off  SenseRad=off  SenseAzim=off  SenseDist=off  SenseInc=off  SenseXDot=on  SenseYDot=on  SenseZDot=on  SenseRadDot=off  SenseAzimDot=off  SenseDistDot=off  SenseIncDot=off  SenseXDDot=off  SenseYDDot=off  SenseZDDot=off  SenseRadDDot=off  SenseAzimDDot=off  SenseDistDDot=off  SenseIncDDot=off
  XForm_WheelRef-to-revolute : sm_lib/Frames and Transforms/Rigid Transform  TranslationMethod=None  TranslationStandardOffset=0  TranslationLengthUnit=m  TranslationStandardAxis=+Z  TranslationCartesianOffset=[0 0 0]  TranslationROffset=0  TranslationROffsetUnits=m  TranslationZOffset=0  TranslationZOffsetUnits=m  TranslationThetaOffset=0  TranslationThetaOffsetUnits=deg  RotationMethod=StandardAxis  RotationAngleUnits=deg  RotationStandardAxis=+X  RotationAngle=-90*sideSign  RotationArbitraryAxis=[0 0 1]  FollAlignAxisA=+Z  BaseAlignAxisA=-Y  FollAlignAxisB=+X  BaseAlignAxisB=+X  RotationSequenceAxes=FollowerAxes  RotationSequence=XYX  RotationSequenceAngles=[0 0 0]  RotationSequenceAnglesUnits=deg  RotationMatrix=[1 0 0; 0 1 0; 0 0 1]
  w - Wheel to Tire transform : MATLAB Function  TreatAsAtomicUnit=on
  Wheel center : PMIOPort  Side=Left
  Gnd : PMIOPort  Port=2  Side=Right
  info : Outport
  wires:
  PS-Simulink Converter1/1 -> Select Fz/1
  Gain/1 -> Simulink-PS Converter6/1
  PS-Simulink Converter/1 -> Camber/1(R), Transpose/1
  PS-Simulink Converter2/1 -> Toe/1(R)
  Toe/1(toe) -> Terminator1/1
  PS-Simulink Converter6/1 -> Vector Concatenate1/1
  PS-Simulink Converter8/1 -> Vector Concatenate1/3
  PS-Simulink Converter7/1 -> Vector Concatenate1/2
  Vector Concatenate1/1 -> Product/2
  V - Wheel to Tire transform/1(y) -> Select Vx/1, Select Vy/1
  PS-Simulink Converter4/1 -> Vector Concatenate2/2
  PS-Simulink Converter5/1 -> Vector Concatenate2/3
  PS-Simulink Converter3/1 -> Vector Concatenate2/1
  Camber/1(IA) -> Camber Sign/1, w - Wheel to Tire transform/1(IA), V - Wheel to Tire transform/1(IA)  "IA"
  Select wz/1 -> Wheel input bus/7  "wz"
  Select Vx/1 -> Wheel input bus/8  "Vx"
  Select Vy/1 -> Wheel input bus/9  "Vy"
  Select Fz/1 -> Dead Zone2/1
  GndZ/1 -> Wheel input bus/4  "GndZ"
  Tire Pressure/1 -> Wheel input bus/3  "Prs"
  AxlTrq/1 -> Wheel input bus/2  "AxlTrq"
  BrkPrs/1 -> Wheel input bus/1  "BrkPrs"
  Wheel input bus/1 -> Wheel input selecto/1
  Combined Slip Wheel 2DOF/2 -> Terminator/1
  Combined Slip Wheel 2DOF/1 -> Bus Selector2/1, info/1, Bus Selector1/1  "Wheel info"
  Bus Selector1/1 -> Gain/1  "<Omega>"
  Bus Selector1/2 -> Add/1  "<z>"
  Bus Selector1/3 -> Add/2  "<Gnd>"
  Bus Selector2/1 -> Camber Sign1/1  "<Gamma>"
  Vector Concatenate3/1 -> F - Tire to Wheel transform/2(u)
  Vector Concatenate4/1 -> M - Tire to Wheel transform/2(u)
  M - Tire to Wheel transform/1(y) -> Simulink-PS Converter2/1
  Constant/1 -> Vector Concatenate3/3
  Lambdas/1 -> Combined Slip Wheel 2DOF/10
  Wheel input selecto/1 -> Combined Slip Wheel 2DOF/1  "<BrkPrs>"
  Wheel input selecto/2 -> Combined Slip Wheel 2DOF/2  "<AxlTrq>"
  Wheel input selecto/3 -> Combined Slip Wheel 2DOF/3  "<Vx>"
  Wheel input selecto/4 -> Combined Slip Wheel 2DOF/4  "<Vy>"
  Wheel input selecto/6 -> Combined Slip Wheel 2DOF/6  "<wz>"
  Wheel input selecto/7 -> Combined Slip Wheel 2DOF/7  "<Prs>"
  Wheel input selecto/8 -> Combined Slip Wheel 2DOF/8  "<GndZ>"
  Wheel input selecto/9 -> Combined Slip Wheel 2DOF/9  "<Fz>"
  Add/1 -> Simulink-PS Converter1/1
  Combined Slip Wheel 2DOF/5 -> Terminator2/1
  Combined Slip Wheel 2DOF/6 -> Vector Concatenate4/1
  Combined Slip Wheel 2DOF/7 -> Vector Concatenate4/2
  Combined Slip Wheel 2DOF/8 -> Vector Concatenate4/3
  Combined Slip Wheel 2DOF/4 -> Dead Zone/1
  Combined Slip Wheel 2DOF/3 -> Dead Zone1/1
  Dead Zone1/1 -> Vector Concatenate3/1
  Dead Zone/1 -> Vector Concatenate3/2
  F - Tire to Wheel transform/1(y) -> Simulink-PS Converter/1
  Camber Sign/1 -> Wheel input bus/6  "IA"
  Product/1 -> V - Wheel to Tire transform/2(u)
  Transpose/1 -> Product/1
  Wheel input selecto/5 -> Combined Slip Wheel 2DOF/5  "<IA>"
  Camber Sign1/1 -> M - Tire to Wheel transform/1(IA), F - Tire to Wheel transform/1(IA)  "IA"
  Dead Zone2/1 -> Wheel input bus/5  "Fz"
  w - Wheel to Tire transform/1(y) -> Select wz/1
  Vector Concatenate2/1 -> w - Wheel to Tire transform/2(u)
  connections:
  Wheel to Contact Patch/LConn1 -- Wheel center/RConn1 -- Connection Label/LConn1 -- XForm_WheelRef-to-revolute/LConn1
  Wheel to Contact Patch/RConn1 -- Gnd contact/RConn1
  Tire/RConn1 -- Inertia/RConn1 -- Wheel revolute/RConn1 -- Rim/RConn1
  Simulink-PS Converter6/RConn1 -- Wheel revolute/LConn2
  Wheel revolute/LConn1 -- XForm_WheelRef-to-revolute/RConn1
  Gnd contact/LConn1 -- Connection Label6/LConn1 -- Gnd/RConn1
  Gnd contact/RConn2 -- PS-Simulink Converter1/LConn1
  Simulink-PS Converter1/RConn1 -- Gnd contact/LConn2
  Connection Label3/LConn1 -- World ref Transform sensor/LConn1
  Connection Label1/LConn1 -- World ref Transform sensor/RConn1
  PS-Simulink Converter/LConn1 -- World ref Transform sensor/RConn2
  Connection Label4/LConn1 -- Transform Sensor1/RConn1
  Connection Label5/LConn1 -- Transform Sensor1/LConn1
  Transform Sensor1/RConn2 -- PS-Simulink Converter2/LConn1
  World ref Transform sensor/RConn6 -- PS-Simulink Converter6/LConn1
  World ref Transform sensor/RConn7 -- PS-Simulink Converter7/LConn1
  World ref Transform sensor/RConn8 -- PS-Simulink Converter8/LConn1
  PS-Simulink Converter3/LConn1 -- World ref Transform sensor/RConn3
  World ref Transform sensor/RConn4 -- PS-Simulink Converter4/LConn1
  PS-Simulink Converter5/LConn1 -- World ref Transform sensor/RConn5
  Simulink-PS Converter2/RConn1 -- External Force and Torque/LConn2
  Simulink-PS Converter/RConn1 -- External Force and Torque/LConn1
  Wheel to Contact Patch - forces/LConn1 -- Connection Label2/LConn1
  Wheel to Contact Patch - forces/RConn1 -- External Force and Torque/RConn1
